simulink model "task8-Simulink"  (R2015b)
settings: Solver=ode23t  StartTime=0.0  StopTime=30  RelTol=1e-3
values from neighbouring files (symbols this model uses):
  A = [0 0 0 1 0 0;     0 0 0 0 1 0;      0 0 0 0 0 1;     (kt-ko)/J1 kt/(J1*n^2) -kt/J1 (dt-do)/J1 dt/(J1*n^2) -dt/J1;    -kt/(Jmg*n^2) -kt/((n^4)*Jmg) kt/((n^2)*Jmg) -dt/(Jmg*n^2) 1/Jmg*(-Km*Kemf/R-dt/(n^4)) dt/(n^2*Jmg);    kt/Jout kt/((n^2)*Jout) (-kt-kr)/Jout dt/Jout dt/((n^2)*Jout) -(dt+dj)/Jout]    [All Tasks Compiled.m]
  B = [0 0 0 0 Km/(R*Jmg) 0]'    [All Tasks Compiled.m]
  C = eye(6)    [All Tasks Compiled.m]
  D = [0 0 0 0 0 0]'    [All Tasks Compiled.m]
  dj = dt    (= 1.5)    [All Tasks Compiled.m]
  kr = kj*(p/(2*pi))^2    [All Tasks Compiled.m]
settings Model: Creator=attalla  LastModifiedBy=daniella.a

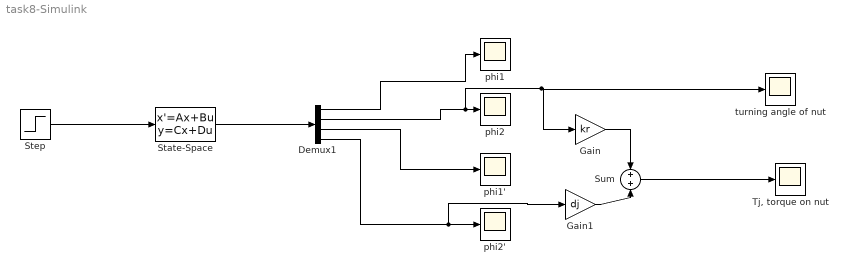
== system task8-Simulink ==
  Demux1 : Demux
  Gain : Gain  Gain=kr
  Gain1 : Gain  Gain=dj
  State-Space : StateSpace  A=A  B=B  C=C  D=D  X0=0
  Step : Step  Time=0  After=24  SampleTime=0
  Sum : Sum
  "Tj, torque on nut" : Scope
  phi1 : Scope
  phi1' : Scope
  "phi2 " : Scope
  phi2' : Scope
  "turning angle of nut " : Scope
  wires:
  Demux1/2 -> "turning angle of nut "/1, Gain/1, "phi2 "/1
  Demux1/3 -> phi1'/1
  Demux1/4 -> Gain1/1, phi2'/1
  Demux1/1 -> phi1/1
  State-Space/1 -> Demux1/1
  Step/1 -> State-Space/1
  Gain/1 -> Sum/1
  Gain1/1 -> Sum/2
  Sum/1 -> "Tj, torque on nut"/1
